simulink library "llc_grc"  (R2024a)
settings: Solver=VariableStepAuto  StartTime=0.0  StopTime=10.0  RelTol=1e-3
undefined symbols (not defined in the file or in its folder): ALLC_volCoolFlowOil_X_degC, ALLC_volCoolFlowWater_X_kW, ALLC_volCoolFlowWater_Y_degC, ALLC_volfCooltFlow_X_degC, CurrM_pwrTMPwrEst_A, EopC_tRrOilTemp_A, LLCM_bTcooltFlowTrig_C, LLCM_tlvtrATemp_C, LLCM_tlvtrBTemp_C, LLCM_tlvtrCTemp_C, LLCM_volfcooltFlowMax_C, LLCM_volfcooltFlowMin_C, LLCM_volfcooltFlowMor_C, LLCM_volfcooltFlowRampDown_C, LLCM_volfcooltFlowRampUp_C, MLLC_volCoolFlowOil_Y_T, MLLC_volCoolFlowWater_Z_M, MLLC_volfCooltFlow_Y_T
libraries: GRC_Lib x3, simulink x2
settings Model: Creator=FVT22063  LastModifiedBy=FVT22063

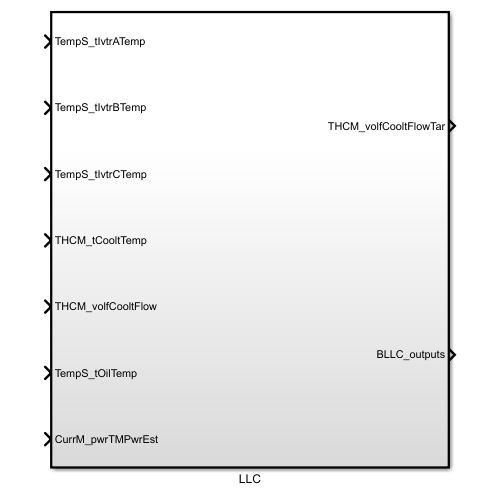
[thumbnail: Simulink's stored preview of the top-level diagram]
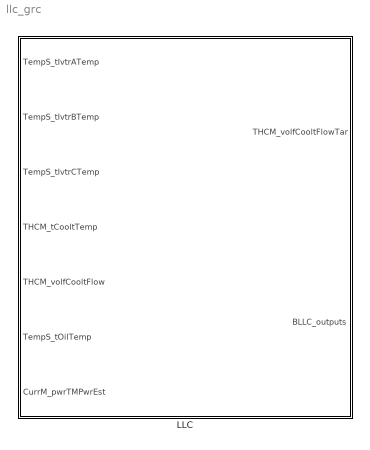
== system llc_grc ==
  LLC : Subsystem  TreatAsAtomicUnit=on
      settings: RTWSystemCode=Nonreusable function  RTWFcnNameOpts=Use subsystem name  RTWFileNameOpts=Use subsystem name

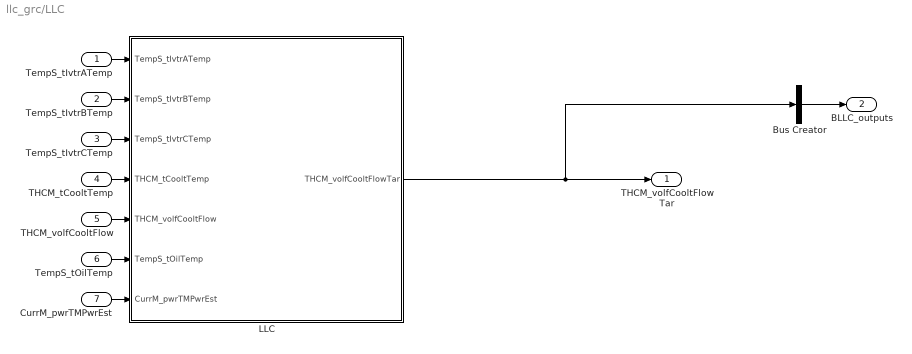
== system llc_grc/LLC ==
  TempS_tIvtrATemp : Inport
  TempS_tIvtrBTemp : Inport  Port=2
  TempS_tIvtrCTemp : Inport  Port=3
  THCM_tCooltTemp : Inport  Port=4
  THCM_volfCooltFlow : Inport  Port=5
  TempS_tOilTemp : Inport  Port=6
  CurrM_pwrTMPwrEst : Inport  Port=7
  Bus Creator : BusCreator  Inputs=1  OutDataTypeStr=Bus: BLLC_outputs  NonVirtualBus=on
  LLC : Subsystem
  THCM_volfCooltFlowTar : Outport
  BLLC_outputs : Outport  Port=2  OutDataTypeStr=Bus: BLLC_outputs
  wires:
  CurrM_pwrTMPwrEst/1 -> LLC/7(CurrM_pwrTMPwrEst)
  TempS_tIvtrCTemp/1 -> LLC/3(TempS_tIvtrCTemp)
  TempS_tIvtrATemp/1 -> LLC/1(TempS_tIvtrATemp)
  TempS_tOilTemp/1 -> LLC/6(TempS_tOilTemp)
  THCM_volfCooltFlow/1 -> LLC/5(THCM_volfCooltFlow)
  LLC/1(THCM_volfCooltFlowTar) -> Bus Creator/1, THCM_volfCooltFlowTar/1
  THCM_tCooltTemp/1 -> LLC/4(THCM_tCooltTemp)
  TempS_tIvtrBTemp/1 -> LLC/2(TempS_tIvtrBTemp)
  Bus Creator/1 -> BLLC_outputs/1

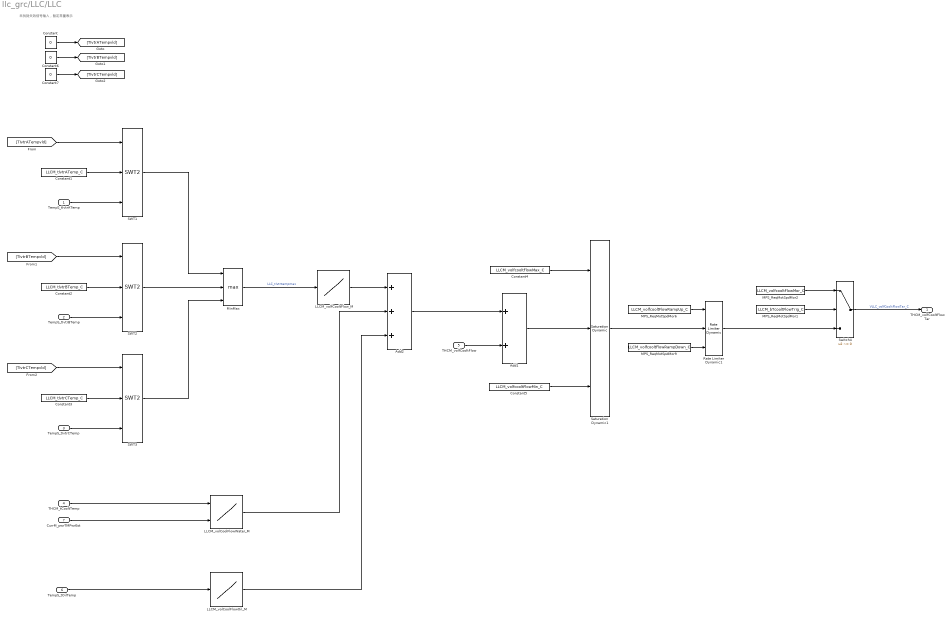
== system llc_grc/LLC/LLC ==
  note: 未找到失效信号输入，暂定常量表示
  TempS_tIvtrATemp : Inport
  TempS_tIvtrBTemp : Inport  Port=2
  TempS_tIvtrCTemp : Inport  Port=3
  THCM_tCooltTemp : Inport  Port=4
  THCM_volfCooltFlow : Inport  Port=5
  TempS_tOilTemp : Inport  Port=6
  CurrM_pwrTMPwrEst : Inport  Port=7
  Add1 : Sum
  Add2 : Sum  Inputs=+++
  Constant : Constant  Value=0
  Constant1 : Constant  Value=LLCM_tlvtrATemp_C
  Constant2 : Constant  Value=LLCM_tlvtrBTemp_C
  Constant3 : Constant  Value=LLCM_tlvtrCTemp_C
  Constant4 : Constant  Value=LLCM_volfcooltFlowMax_C
  Constant5 : Constant  Value=LLCM_volfcooltFlowMin_C
  Constant6 : Constant  Value=0
  Constant7 : Constant  Value=0
  LLCM_volCoolFlowOil_M : Lookup_n-D  NumberOfTableDimensions=1  BreakpointsForDimension1=ALLC_volCoolFlowOil_X_degC  BreakpointsForDimension2=CurrM_pwrTMPwrEst_A  Table=MLLC_volCoolFlowOil_Y_T  ExtrapMethod=Clip  UseLastTableValue=on  InternalRulePriority=Speed  RndMeth=Simplest
  LLCM_volCoolFlowWater_M : Lookup_n-D  BreakpointsForDimension1=ALLC_volCoolFlowWater_Y_degC  BreakpointsForDimension2=ALLC_volCoolFlowWater_X_kW  Table=MLLC_volCoolFlowWater_Z_M  ExtrapMethod=Clip  UseLastTableValue=on  InternalRulePriority=Speed  RndMeth=Simplest
      settings: InputPortMap=u0,u1
  LLCM_volfCooltFlow_M : Lookup_n-D  NumberOfTableDimensions=1  BreakpointsForDimension1=ALLC_volfCooltFlow_X_degC  BreakpointsForDimension2=EopC_tRrOilTemp_A  Table=MLLC_volfCooltFlow_Y_T  ExtrapMethod=Clip  UseLastTableValue=on  InternalRulePriority=Speed  RndMeth=Simplest
  MPS_ReqMotSpdMor1 : Constant  Value=LLCM_bTcooltFlowTrig_C
  MPS_ReqMotSpdMor2 : Constant  Value=LLCM_volfcooltFlowMor_C
  MPS_ReqMotSpdMor6 : Constant  Value=LLCM_volfcooltFlowRampUp_C
  MPS_ReqMotSpdMor9 : Constant  Value=LLCM_volfcooltFlowRampDown_C
  MinMax : MinMax  Function=max  Inputs=3
  Rate Limiter Dynamic1 : simulink/Discontinuities/Rate Limiter Dynamic
  SWT1 : GRC_Lib/SignalSwitch/SWT2  OpDT=double
  SWT2 : GRC_Lib/SignalSwitch/SWT2  OpDT=double
  SWT3 : GRC_Lib/SignalSwitch/SWT2  OpDT=double
  Saturation Dynamic1 : simulink/Discontinuities/Saturation Dynamic  OutMin=[]  OutMax=[]  OutDataTypeStr=Inherit: Same as second input  OutDataType=fixdt(1, 16)  OutScaling=2^-10  DoSatur=off
  Switch4 : Switch  Criteria=u2 ~= 0  SaturateOnIntegerOverflow=off  InputSameDT=off
  THCM_volfCooltFlowTar : Outport  VectorParamsAs1DForOutWhenUnconnected=off
  wires:
  Constant6/1 -> [TIvtrBTempvld]
  SWT2/1 -> MinMax/2
  LLCM_volCoolFlowWater_M/1 -> Add2/2
  Add1/1 -> Saturation Dynamic1/2
  Constant2/1 -> SWT2/2
  Constant/1 -> [TIvtrATempvld]
  TempS_tOilTemp/1 -> LLCM_volCoolFlowOil_M/1
  TempS_tIvtrATemp/1 -> SWT1/3
  MinMax/1 -> LLCM_volfCooltFlow_M/1  "LLC_tIvtrtempmax"
  Constant3/1 -> SWT3/2
  Constant7/1 -> [TIvtrCTempvld]
  TempS_tIvtrBTemp/1 -> SWT2/3
  Add2/1 -> Add1/1
  TempS_tIvtrCTemp/1 -> SWT3/3
  Constant1/1 -> SWT1/2
  Switch4/1 -> THCM_volfCooltFlowTar/1  "VLLC_volfCooltFlowTar_C"
  MPS_ReqMotSpdMor9/1 -> Rate Limiter Dynamic1/3
  Saturation Dynamic1/1 -> Rate Limiter Dynamic1/2
  Rate Limiter Dynamic1/1 -> Switch4/3
  THCM_tCooltTemp/1 -> LLCM_volCoolFlowWater_M/1
  [TIvtrBTempvld] -> SWT2/1
  LLCM_volCoolFlowOil_M/1 -> Add2/3
  Constant5/1 -> Saturation Dynamic1/3
  MPS_ReqMotSpdMor1/1 -> Switch4/2
  MPS_ReqMotSpdMor6/1 -> Rate Limiter Dynamic1/1
  SWT1/1 -> MinMax/1
  Constant4/1 -> Saturation Dynamic1/1
  LLCM_volfCooltFlow_M/1 -> Add2/1
  [TIvtrCTempvld] -> SWT3/1
  MPS_ReqMotSpdMor2/1 -> Switch4/1
  CurrM_pwrTMPwrEst/1 -> LLCM_volCoolFlowWater_M/2
  SWT3/1 -> MinMax/3
  [TIvtrATempvld] -> SWT1/1
  THCM_volfCooltFlow/1 -> Add1/2
